simulink library "elementsLibrary"  (R2018a)
settings: Solver=VariableStepAuto  StartTime=0.0  StopTime=10.0  RelTol=1e-3
undefined symbols (not defined in the file): aerodynamics, ascent, avionics, environment, payload, propulsion, pvessel, recovery, rocket, sequencer
libraries: snippetLibrary x43, $bdroot x24, sharedutil x8, theirs_elementsLibrary x3, simulink_extras x1, aerolibutil x1
(part 4 of 4)

== system elementsLibrary/barrowmanExt/Coefficient of normal force/Body tube correction ==
  AOA : Inport
  Constant : Constant  Value=aerodynamics.K
  Constant1 : Constant  Value=aerodynamics.Ap
  Constant2 : Constant  Value=aerodynamics.Ar
  Divide : Product  Inputs=***/
  Sin : Trigonometry
  Square : Math  Operator=square  SaturateOnIntegerOverflow=on
  Cn_BodyCorrection : Outport
  wires:
  AOA/1 -> Sin/1
  Sin/1 -> Square/1
  Constant2/1 -> Divide/4
  Constant/1 -> Divide/1
  Constant1/1 -> Divide/2
  Square/1 -> Divide/3
  Divide/1 -> Cn_BodyCorrection/1

== system elementsLibrary/barrowmanExt/Coefficient of normal force/Cna Body Tube ==
  AOA : Inport
  Constant1 : Constant  Value=2
  Multiply : Product
  Subsystem : Subsystem
  Cna_nosecone : Outport
  wires:
  AOA/1 -> Subsystem/1(AOA)
  Subsystem/1(Correction) -> Multiply/2
  Constant1/1 -> Multiply/1
  Multiply/1 -> Cna_nosecone/1

== system elementsLibrary/barrowmanExt/Coefficient of normal force/Cna Fins ==
  AOA : Inport
  Mach : Inport  Port=2
  k1 : Inport  Port=3
  k2 : Inport  Port=4
  k3 : Inport  Port=5
  Constant : Constant  Value=aerodynamics.nf/2
  Constant1 : Constant  Value=aerodynamics.K_BF
  If : If  IfExpression=u1 <= 0.9  ElseIfExpressions=u1 >= 1.5
  Merge : Merge  Inputs=3
  Multiply : Product
  Multiply1 : Product
  Supersonic case : Subsystem  TreatAsAtomicUnit=on
  Transonic case : Subsystem  TreatAsAtomicUnit=on
  subsonic case : Subsystem  TreatAsAtomicUnit=on
  Cna_fins_w_FB_inter : Outport
  wires:
  Mach/1 -> Transonic case/1(Mach), subsonic case/1(Mach), If/1
  If/1 -> subsonic case/Action
  AOA/1 -> Supersonic case/1(AOA)
  k1/1 -> Supersonic case/2(k1)
  k2/1 -> Supersonic case/3(k2)
  k3/1 -> Supersonic case/4(k3)
  If/2 -> Supersonic case/Action
  If/3 -> Transonic case/Action
  Merge/1 -> Multiply/2
  Constant/1 -> Multiply/1
  subsonic case/1(Cna_1fin_subsonic) -> Merge/1
  Transonic case/1(Cna_1fin_Transonic) -> Merge/2
  Supersonic case/1(Cna_1fin_supersonic) -> Merge/3
  Constant1/1 -> Multiply1/1
  Multiply/1 -> Multiply1/2
  Multiply1/1 -> Cna_fins_w_FB_inter/1

== system elementsLibrary/barrowmanExt/Moment Coefficients from nosetip/Pitch Moment Coeff ==
  Xcp : Inport
  Cn : Inport  Port=2
  Constant : Constant  Value=aerodynamics.dn
  Divide : Product  Inputs=**/
  Cm_pitch_cp : Outport
  wires:
  Xcp/1 -> Divide/1
  Cn/1 -> Divide/2
  Constant/1 -> Divide/3
  Divide/1 -> Cm_pitch_cp/1

== system elementsLibrary/barrowmanExt/Moment Coefficients from nosetip/Subsystem ==
  Cm_pitch_cp : Inport
  Cn : Inport  Port=2
  Xcg : Inport  Port=3
  Constant : Constant  Value=aerodynamics.dn
  Divide : Product  Inputs=**/
  Subtract : Sum  Inputs=+-
  Cm_pitch_cg : Outport
  wires:
  Cn/1 -> Divide/1
  Xcg/1 -> Divide/2
  Constant/1 -> Divide/3
  Cm_pitch_cp/1 -> Subtract/1
  Divide/1 -> Subtract/2
  Subtract/1 -> Cm_pitch_cg/1

== system elementsLibrary/Ascentv1/Calculate Aero Coeffs & Center of Pressure/calculate ZAOA_cd/BaseCd ==
  Cd_fb : Inport
  Constant : Constant  Value=ascent.aerodynamics.dd
  Constant1 : Constant  Value=ascent.aerodynamics.db
  Constant2 : Constant  Value=3
  Divide : Product  Inputs=*/
  Divide1 : Product  Inputs=*/
  Gain : Gain  Gain=0.029
  Power : Math  Operator=pow  SaturateOnIntegerOverflow=on
  Sqrt : Sqrt  SaturateOnIntegerOverflow=on
  Cdb : Outport
  wires:
  Cd_fb/1 -> Sqrt/1
  Constant1/1 -> Divide/2
  Constant/1 -> Divide/1
  Divide/1 -> Power/1
  Constant2/1 -> Power/2
  Power/1 -> Divide1/1
  Sqrt/1 -> Divide1/2
  Divide1/1 -> Gain/1
  Gain/1 -> Cdb/1

== system elementsLibrary/Ascentv1/Calculate Aero Coeffs & Center of Pressure/calculate ZAOA_cd/FinsetCd ==
  Cf_f : Inport
  Add : Sum
  Constant : Constant  Value=ascent.aerodynamics.A_fp
  Constant1 : Constant  Value=ascent.aerodynamics.df
  Constant2 : Constant
  Constant3 : Constant  Value=ascent.aerodynamics.tf
  Constant4 : Constant  Value=ascent.aerodynamics.lm
  Divide : Product  Inputs=*/
  Divide1 : Product  Inputs=*/
  Gain : Gain  Gain=4
  Gain1 : Gain  Gain=pi
  Gain2 : Gain  Gain=2
  Gain3 : Gain  Gain=2
  Gain4 : Gain  Gain=ascent.aerodynamics.nf
  Multiply : Product  Inputs=3
  Square : Math  Operator=square  SaturateOnIntegerOverflow=on
  Cdf : Outport
  wires:
  Constant/1 -> Gain/1
  Constant1/1 -> Square/1
  Gain1/1 -> Divide/2
  Divide/1 -> Multiply/3
  Square/1 -> Gain1/1
  Cf_f/1 -> Gain2/1
  Constant2/1 -> Add/1
  Constant3/1 -> Divide1/1
  Constant4/1 -> Divide1/2
  Divide1/1 -> Gain3/1
  Gain3/1 -> Add/2
  Add/1 -> Multiply/2
  Gain2/1 -> Multiply/1
  Gain4/1 -> Divide/1
  Gain/1 -> Gain4/1
  Multiply/1 -> Cdf/1

== system elementsLibrary/Ascentv1/Calculate Aero Coeffs & Center of Pressure/calculate ZAOA_cd/ForebodyCd ==
  Cf_fb : Inport
  Add : Sum  Inputs=+++
  Add1 : Sum  Inputs=+++
  Constant : Constant
  Constant1 : Constant  Value=60
  Constant2 : Constant  Value=ascent.aerodynamics.lb/ascent.aerodynamics.db
  Constant3 : Constant  Value=ascent.aerodynamics.l_TR/ascent.aerodynamics.db
  Constant4 : Constant  Value=3
  Constant5 : Constant  Value=1-(ascent.aerodynamics.dd/ascent.aerodynamics.db)
  Constant6 : Constant  Value=ascent.aerodynamics.lc/ascent.aerodynamics.db
  Constant7 : Constant  Value=ascent.aerodynamics.ln/ascent.aerodynamics.db
  Constant8 : Constant  Value=ascent.aerodynamics.lb/ascent.aerodynamics.db
  Divide : Product  Inputs=/*
  Gain : Gain  Gain=0.0025
  Gain1 : Gain  Gain=2
  Gain2 : Gain  Gain=2.7
  Gain3 : Gain  Gain=4
  Multiply : Product  Inputs=3
  Multiply1 : Product
  Power : Math  Operator=pow  SaturateOnIntegerOverflow=on
  Cd_fb : Outport
  wires:
  Multiply/1 -> Cd_fb/1
  Cf_fb/1 -> Multiply/1
  Add/1 -> Multiply/2
  Add1/1 -> Multiply/3
  Constant/1 -> Add/3
  Divide/1 -> Add/1
  Constant1/1 -> Divide/2
  Gain/1 -> Add/2
  Constant2/1 -> Gain/1
  Power/1 -> Divide/1
  Constant3/1 -> Power/1
  Constant4/1 -> Power/2
  Gain1/1 -> Add1/1
  Multiply1/1 -> Gain1/1
  Constant5/1 -> Multiply1/1
  Constant6/1 -> Multiply1/2
  Gain2/1 -> Add1/2
  Gain3/1 -> Add1/3
  Constant7/1 -> Gain2/1
  Constant8/1 -> Gain3/1

== system elementsLibrary/Ascentv1/Calculate Aero Coeffs & Center of Pressure/calculate ZAOA_cd/InterferenceCd ==
  Cf_f : Inport
  Add : Sum
  Constant : Constant  Value=ascent.aerodynamics.A_fp - ascent.aerodynamics.A_fe
  Constant1 : Constant  Value=ascent.aerodynamics.df
  Constant2 : Constant
  Constant3 : Constant  Value=ascent.aerodynamics.tf
  Constant4 : Constant  Value=ascent.aerodynamics.lm
  Divide : Product  Inputs=*/
  Divide1 : Product  Inputs=*/
  Gain : Gain  Gain=4
  Gain1 : Gain  Gain=pi
  Gain2 : Gain  Gain=2
  Gain3 : Gain  Gain=2
  Gain4 : Gain  Gain=ascent.aerodynamics.nf
  Multiply : Product  Inputs=3
  Square : Math  Operator=square  SaturateOnIntegerOverflow=on
  Cdi : Outport
  wires:
  Add/1 -> Multiply/2
  Multiply/1 -> Cdi/1
  Square/1 -> Gain1/1
  Constant1/1 -> Square/1
  Constant/1 -> Gain/1
  Gain1/1 -> Divide/2
  Divide/1 -> Multiply/3
  Constant2/1 -> Add/1
  Gain4/1 -> Divide/1
  Constant4/1 -> Divide1/2
  Divide1/1 -> Gain3/1
  Gain3/1 -> Add/2
  Gain2/1 -> Multiply/1
  Constant3/1 -> Divide1/1
  Gain/1 -> Gain4/1
  Cf_f/1 -> Gain2/1

== system elementsLibrary/Ascentv2/Rotational/Inertia_Matrix /parallelAxisTheo_restricted ==
  emptyInertia : Inport
  motorInertias : Inport  Port=2
  propellantMass : Inport  Port=3
  rocketEmptyXcg : Inport  Port=4
  motorProperties : Inport  Port=5
  Add : Sum
  Add1 : Sum
  Add2 : Sum
  Bus Selector : BusSelector  OutputSignals=x_gm_B,x_cg_B
  Constant{1..7} (7 alike) : Constant  Value=0
  Create 3x3 Matrix : sharedutil/Create 3x3 Matrix  aMode=aMode
  Multiply : Product
  Square : Math  Operator=square  SaturateOnIntegerOverflow=on
  Subtract : Sum  Inputs=+-
  J_rocket : Outport
  wires:
  Constant6/1 -> Create 3x3 Matrix/7
  Constant7/1 -> Create 3x3 Matrix/4
  Create 3x3 Matrix/1 -> Add1/2
  Constant4/1 -> Create 3x3 Matrix/6
  Constant5/1 -> Create 3x3 Matrix/8
  Constant1/1 -> Create 3x3 Matrix/2
  Multiply/1 -> Create 3x3 Matrix/5, Create 3x3 Matrix/9
  Constant2/1 -> Create 3x3 Matrix/3
  Add/1 -> J_rocket/1  "J_equivalent"
  Add1/1 -> Add/2
  propellantMass/1 -> Multiply/1
  motorInertias/1 -> Add1/1
  emptyInertia/1 -> Add/1
  rocketEmptyXcg/1 -> Subtract/2
  Constant3/1 -> Create 3x3 Matrix/1
  Subtract/1 -> Square/1
  Square/1 -> Multiply/2
  Bus Selector/1 -> Add2/1  "<x_gm_B>"
  Bus Selector/2 -> Add2/2  "<x_cg_B>"
  Add2/1 -> Subtract/1
  motorProperties/1 -> Bus Selector/1

== system elementsLibrary/HREV1/Chamber_Ballistics/calc_chamber_params/If Action Subsystem ==
  In1 : Inport
  Action Port : ActionPort  ActionType=then
  Out1 : Outport
  wires:
  In1/1 -> Out1/1

== system elementsLibrary/HREV1/Chamber_Ballistics/calc_chamber_params/If Action Subsystem1 ==
  In1 : Inport
  Action Port : ActionPort  ActionType=else
  Out1 : Outport
  wires:
  In1/1 -> Out1/1

== system elementsLibrary/HREV1/Chamber_Ballistics/calc_chamber_params/calc_Tc ==
  OF_ratio : Inport
  Add : Sum  Inputs=+++++
  Constant : Constant  Value=-15.854
  Constant1 : Constant  Value=4
  Constant2 : Constant  Value=314.21
  Constant3 : Constant  Value=3
  Constant4 : Constant  Value=-2334.4
  Constant5 : Constant  Value=2
  Constant6 : Constant  Value=-5742.5
  Constant7 : Constant  Value=7623.5
  Multiply{,1..3} (4 alike) : Product
  Power1 : Math  Operator=pow  SaturateOnIntegerOverflow=on
  Power2 : Math  Operator=pow  SaturateOnIntegerOverflow=on
  Power3 : Math  Operator=pow  SaturateOnIntegerOverflow=on
  Saturation : Saturate  UpperLimit=10000  LowerLimit=273.15
  Tc : Outport
  wires:
  OF_ratio/1 -> Power3/1, Power1/1, Power2/1, Multiply3/2
  Multiply/1 -> Add/1
  Multiply1/1 -> Add/2
  Multiply2/1 -> Add/3
  Multiply3/1 -> Add/4
  Constant6/1 -> Add/5
  Power3/1 -> Multiply2/2
  Power2/1 -> Multiply/2
  Power1/1 -> Multiply1/2
  Constant/1 -> Multiply/1
  Constant1/1 -> Power2/2
  Constant2/1 -> Multiply1/1
  Constant3/1 -> Power1/2
  Constant4/1 -> Multiply2/1
  Constant5/1 -> Power3/2
  Constant7/1 -> Multiply3/1
  Saturation/1 -> Tc/1
  Add/1 -> Saturation/1

== system elementsLibrary/HREV1/Chamber_Ballistics/calc_mdot_fuel/calc_OF ==
  mdot_fuel : Inport
  mdot_oxi : Inport  Port=2
  Constant : Constant  Value=0
  Divide : Product  Inputs=*/
  If : If
  If Action Subsystem : Subsystem  TreatAsAtomicUnit=on
  If Action Subsystem1 : Subsystem  TreatAsAtomicUnit=on
  Merge : Merge
  OF_ratio : Outport
  wires:
  mdot_oxi/1 -> Divide/1
  mdot_fuel/1 -> If/1, Divide/2
  If Action Subsystem1/1(Out1) -> Merge/2
  Constant/1 -> If Action Subsystem1/1(In1)
  If/2 -> If Action Subsystem1/Action
  If Action Subsystem/1(Out1) -> Merge/1
  If/1 -> If Action Subsystem/Action
  Merge/1 -> OF_ratio/1
  Divide/1 -> If Action Subsystem/1(In1)

== system elementsLibrary/HREV1/Chamber_Ballistics/calc_mdot_fuel/calc_massFlux_oxi ==
  Dp : Inport
  mdot_oxi : Inport  Port=2
  Divide : Product  Inputs=*/
  Gain : Gain  Gain=4
  Multiply : Product
  Pi : Constant  Value=pi
  Square : Math  Operator=square  SaturateOnIntegerOverflow=on
  Gox : Outport
  wires:
  Divide/1 -> Gox/1
  Dp/1 -> Square/1
  Multiply/1 -> Divide/2
  Square/1 -> Multiply/2
  Pi/1 -> Multiply/1
  Gain/1 -> Divide/1
  mdot_oxi/1 -> Gain/1

== system elementsLibrary/HREV1/Chamber_Ballistics/calc_mdot_fuel/calc_mdot_fuel ==
  rdot_fuel : Inport
  Dp : Inport  Port=2
  rho_oxi : Inport  Port=3
  Add : Sum  Inputs=-+
  Constant : Constant  Value=0
  Constant1 : Constant  Value=propulsion.initMassFuel
  Integrator : Integrator
  LessThanOrEqual : RelationalOperator  Operator=>  OutDataTypeStr=boolean  RndMeth=Simplest
  Multiply : Product  Inputs=5
  Multiply1 : Product
  Pi : Constant  Value=pi
  grainL : Constant  Value=propulsion.Lfg
  mdot_fuel : Outport
  massFuel : Outport  Port=2
  wires:
  Multiply/1 -> Multiply1/1
  rho_oxi/1 -> Multiply/1
  Pi/1 -> Multiply/2
  rdot_fuel/1 -> Multiply/5
  Dp/1 -> Multiply/3
  grainL/1 -> Multiply/4
  Integrator/1 -> Add/1
  Constant1/1 -> Add/2
  Add/1 -> massFuel/1, LessThanOrEqual/1
  Constant/1 -> LessThanOrEqual/2
  LessThanOrEqual/1 -> Multiply1/2
  Multiply1/1 -> Integrator/1, mdot_fuel/1

== system elementsLibrary/HREV1/Chamber_Ballistics/calc_mdot_fuel/calc_rdot_fuel ==
  Gox : Inport
  Multiply : Product
  Power : Math  Operator=pow  SaturateOnIntegerOverflow=on
  a : Constant  Value=propulsion.a
  mm/s_to_m/s : Gain  Gain=0.001
  n : Constant  Value=propulsion.n
  rdot_fuel : Outport
  wires:
  Multiply/1 -> mm/s_to_m/s/1
  Power/1 -> Multiply/2
  Gox/1 -> Power/1
  n/1 -> Power/2
  a/1 -> Multiply/1
  mm/s_to_m/s/1 -> rdot_fuel/1

== system elementsLibrary/SingleChute/Rotational Motion/equations of rotational motion/invInertia_Matrix_P ==
  Constant : Constant  Value=recovery.inertiaMatP(1,1)
  Constant1 : Constant  Value=recovery.inertiaMatP(1,2)
  Constant2 : Constant  Value=recovery.inertiaMatP(1,3)
  Constant3 : Constant  Value=recovery.inertiaMatP(2,1)
  Constant4 : Constant  Value=recovery.inertiaMatP(2,2)
  Constant5 : Constant  Value=recovery.inertiaMatP(2,3)
  Constant6 : Constant  Value=recovery.inertiaMatP(3,1)
  Constant7 : Constant  Value=recovery.inertiaMatP(3,2)
  Constant8 : Constant  Value=recovery.inertiaMatP(3,3)
  Create 3x3 Matrix : sharedutil/Create 3x3 Matrix  aMode=aMode
  inverse_3x3 : snippetLibrary/mathSnippets/inverse_3x3
  invInerMat : Outport
  inerMat : Outport  Port=2
  wires:
  Constant3/1 -> Create 3x3 Matrix/4
  Constant8/1 -> Create 3x3 Matrix/9
  Create 3x3 Matrix/1 -> inerMat/1, inverse_3x3/1
  Constant4/1 -> Create 3x3 Matrix/5
  inverse_3x3/1 -> invInerMat/1
  Constant/1 -> Create 3x3 Matrix/1
  Constant5/1 -> Create 3x3 Matrix/6
  Constant7/1 -> Create 3x3 Matrix/8
  Constant1/1 -> Create 3x3 Matrix/2
  Constant2/1 -> Create 3x3 Matrix/3
  Constant6/1 -> Create 3x3 Matrix/7

== system elementsLibrary/SingleChute/Rotational Motion/equations of rotational motion/invInertia_Matrix_R ==
  Constant : Constant  Value=recovery.inertiaMatR(1,1)
  Constant1 : Constant  Value=recovery.inertiaMatR(1,2)
  Constant2 : Constant  Value=recovery.inertiaMatR(1,3)
  Constant3 : Constant  Value=recovery.inertiaMatR(2,1)
  Constant4 : Constant  Value=recovery.inertiaMatR(2,2)
  Constant5 : Constant  Value=recovery.inertiaMatR(2,3)
  Constant6 : Constant  Value=recovery.inertiaMatR(3,1)
  Constant7 : Constant  Value=recovery.inertiaMatR(3,2)
  Constant8 : Constant  Value=recovery.inertiaMatR(3,3)
  Create 3x3 Matrix : sharedutil/Create 3x3 Matrix  aMode=aMode
  inverse_3x3 : snippetLibrary/mathSnippets/inverse_3x3
  invInerMat : Outport
  inerMat : Outport  Port=2
  wires:
  inverse_3x3/1 -> invInerMat/1
  Constant4/1 -> Create 3x3 Matrix/5
  Constant2/1 -> Create 3x3 Matrix/3
  Constant7/1 -> Create 3x3 Matrix/8
  Constant/1 -> Create 3x3 Matrix/1
  Constant1/1 -> Create 3x3 Matrix/2
  Constant5/1 -> Create 3x3 Matrix/6
  Constant3/1 -> Create 3x3 Matrix/4
  Constant6/1 -> Create 3x3 Matrix/7
  Constant8/1 -> Create 3x3 Matrix/9
  Create 3x3 Matrix/1 -> inerMat/1, inverse_3x3/1

== system elementsLibrary/barrowmanExt/Center of Pressure/Calc Xcp fins/If Action Subsystem ==
  Action Port : ActionPort
  Constant : Constant  Value=aerodynamics.Xcp_fins
  Xcp_fins_subMach0.5 : Outport
  wires:
  Constant/1 -> Xcp_fins_subMach0.5/1

== system elementsLibrary/barrowmanExt/Center of Pressure/Calc Xcp fins/If Action Subsystem1 ==
  Mach : Inport
  Action Port : ActionPort
  Add : Sum
  Calc Beta : Subsystem
  Constant : Constant  Value=aerodynamics.AsRa
  Constant1 : Constant  Value=aerodynamics.lm
  Constant2 : Constant  Value=0.67
  Constant3 : Constant  Value=2*aerodynamics.AsRa
  Constant4 : Constant
  Constant5 : Constant  Value=aerodynamics.macLead
  Divide : Product  Inputs=**/
  Multiply : Product
  Multiply1 : Product
  Subtract : Sum  Inputs=+-
  Subtract1 : Sum  Inputs=+-
  Xcp_fins_above2 : Outport
  wires:
  Mach/1 -> Calc Beta/1(Mach)
  Calc Beta/1(Beta) -> Multiply1/1, Multiply/2
  Constant/1 -> Multiply/1
  Multiply/1 -> Subtract/1
  Constant2/1 -> Subtract/2
  Constant3/1 -> Multiply1/2
  Multiply1/1 -> Subtract1/1
  Constant4/1 -> Subtract1/2
  Subtract1/1 -> Divide/3
  Subtract/1 -> Divide/2
  Constant1/1 -> Divide/1
  Divide/1 -> Add/2
  Constant5/1 -> Add/1
  Add/1 -> Xcp_fins_above2/1

== system elementsLibrary/barrowmanExt/Center of Pressure/Calc Xcp fins/If Action Subsystem2 ==
  Mach : Inport
  Action Port : ActionPort
  Add : Sum
  Constant : Constant  Value=aerodynamics.macLead
  Polynomial : Polyval  Coefs=aerodynamics.finXcpPoly
  Xcp_finsTrans : Outport
  wires:
  Mach/1 -> Polynomial/1
  Polynomial/1 -> Add/1
  Constant/1 -> Add/2
  Add/1 -> Xcp_finsTrans/1

== system elementsLibrary/barrowmanExt/Coefficent of drag 0 AOA/Pressure Drag Coefficient/Fin Pressure Drag ==
  stagD : Inport
  baseD : Inport  Port=2
  Add : Sum
  Atan2 : Trigonometry  Operator=atan2
  Constant : Constant  Value=aerodynamics.lw
  Constant1 : Constant  Value=aerodynamics.nf
  Constant2 : Constant  Value=aerodynamics.tf
  Constant3 : Constant  Value=aerodynamics.Ar
  Constant4 : Constant  Value=aerodynamics.lw
  Constant5 : Constant  Value=aerodynamics.ls
  Cos : Trigonometry  Operator=cos
  Divide : Product  Inputs=*/
  Multiply : Product
  Multiply1 : Product  Inputs=4
  Square : Math  Operator=square  SaturateOnIntegerOverflow=on
  finPD : Outport
  wires:
  Square/1 -> Multiply/1
  Cos/1 -> Square/1
  Atan2/1 -> Cos/1
  Constant4/1 -> Atan2/2
  Constant5/1 -> Atan2/1
  Divide/1 -> finPD/1
  Constant3/1 -> Divide/2
  Multiply1/1 -> Divide/1
  Constant2/1 -> Multiply1/4
  Constant1/1 -> Multiply1/3
  Constant/1 -> Multiply1/2
  Add/1 -> Multiply1/1
  Multiply/1 -> Add/1
  baseD/1 -> Add/2
  stagD/1 -> Multiply/2

== system elementsLibrary/barrowmanExt/Coefficient of normal force/Cna Body Tube/Subsystem ==
  AOA : Inport
  If : If  IfExpression=u1 < 0.0001
  If Action Subsystem : Subsystem  TreatAsAtomicUnit=on
  If Action Subsystem1 : Subsystem  TreatAsAtomicUnit=on
  Merge : Merge
  Correction : Outport
  wires:
  AOA/1 -> If Action Subsystem1/1(AOA), If/1
  If/1 -> If Action Subsystem/Action
  If/2 -> If Action Subsystem1/Action
  If Action Subsystem/1(Correction) -> Merge/1
  If Action Subsystem1/1(Correction) -> Merge/2
  Merge/1 -> Correction/1

== system elementsLibrary/barrowmanExt/Coefficient of normal force/Cna Fins/Supersonic case ==
  AOA : Inport
  k1 : Inport  Port=2
  k2 : Inport  Port=3
  k3 : Inport  Port=4
  Action Port : ActionPort
  Single Fin Cna Supersonic : Subsystem
  Cna_1fin_supersonic : Outport
  wires:
  AOA/1 -> Single Fin Cna Supersonic/1(AOA)
  k1/1 -> Single Fin Cna Supersonic/2(k1)
  k3/1 -> Single Fin Cna Supersonic/4(k3)
  k2/1 -> Single Fin Cna Supersonic/3(k2)
  Single Fin Cna Supersonic/1(Cna_1fin_supersonic) -> Cna_1fin_supersonic/1

== system elementsLibrary/barrowmanExt/Coefficient of normal force/Cna Fins/Transonic case ==
  Mach : Inport
  Action Port : ActionPort
  1-D Lookup Table : Lookup_n-D  NumberOfTableDimensions=1  BreakpointsForDimension1=aerodynamics.transCnaFinsBreakpoints  Table=aerodynamics.transCnaFins  InternalRulePriority=Speed  RndMeth=Simplest  InputSameDT=on
  Cna_1fin_Transonic : Outport
  wires:
  Mach/1 -> 1-D Lookup Table/1
  1-D Lookup Table/1 -> Cna_1fin_Transonic/1

== system elementsLibrary/barrowmanExt/Coefficient of normal force/Cna Fins/subsonic case ==
  Mach : Inport
  Action Port : ActionPort
  Single Fin Cna subsonic : Subsystem
  Cna_1fin_subsonic : Outport
  wires:
  Mach/1 -> Single Fin Cna subsonic/1(Mach)
  Single Fin Cna subsonic/1(Cna_1Fin_subsonic) -> Cna_1fin_subsonic/1

== system elementsLibrary/HREV1/Chamber_Ballistics/calc_mdot_fuel/calc_OF/If Action Subsystem ==
  In1 : Inport
  Action Port : ActionPort  ActionType=then
  Out1 : Outport
  wires:
  In1/1 -> Out1/1

== system elementsLibrary/HREV1/Chamber_Ballistics/calc_mdot_fuel/calc_OF/If Action Subsystem1 ==
  In1 : Inport
  Action Port : ActionPort  ActionType=else
  Out1 : Outport
  wires:
  In1/1 -> Out1/1

== system elementsLibrary/barrowmanExt/Center of Pressure/Calc Xcp fins/If Action Subsystem1/Calc Beta ==
  Mach : Inport
  Abs : Abs
  Constant : Constant
  Sqrt : Sqrt  SaturateOnIntegerOverflow=on
  Square : Math  Operator=square  SaturateOnIntegerOverflow=on
  Subtract : Sum  Inputs=+-
  Beta : Outport
  wires:
  Mach/1 -> Square/1
  Constant/1 -> Subtract/2
  Square/1 -> Subtract/1
  Subtract/1 -> Abs/1
  Abs/1 -> Sqrt/1
  Sqrt/1 -> Beta/1

== system elementsLibrary/barrowmanExt/Coefficient of normal force/Cna Body Tube/Subsystem/If Action Subsystem ==
  Action Port : ActionPort
  Constant : Constant
  Correction : Outport
  wires:
  Constant/1 -> Correction/1

== system elementsLibrary/barrowmanExt/Coefficient of normal force/Cna Body Tube/Subsystem/If Action Subsystem1 ==
  AOA : Inport
  Action Port : ActionPort
  Divide : Product  Inputs=*/
  Sin : Trigonometry
  Correction : Outport
  wires:
  AOA/1 -> Divide/2, Sin/1
  Sin/1 -> Divide/1
  Divide/1 -> Correction/1

== system elementsLibrary/barrowmanExt/Coefficient of normal force/Cna Fins/Supersonic case/Single Fin Cna Supersonic ==
  AOA : Inport
  k1 : Inport  Port=2
  k2 : Inport  Port=3
  k3 : Inport  Port=4
  Add : Sum  Inputs=+++
  Constant : Constant  Value=aerodynamics.A_fwt/aerodynamics.Ar
  Multiply : Product
  Multiply1 : Product
  Multiply2 : Product
  Square : Math  Operator=square  SaturateOnIntegerOverflow=on
  Cna_1fin_supersonic : Outport
  wires:
  AOA/1 -> Square/1, Multiply/2
  Square/1 -> Multiply1/1
  k3/1 -> Multiply1/2
  k2/1 -> Multiply/1
  Multiply1/1 -> Add/3
  Multiply/1 -> Add/2
  k1/1 -> Add/1
  Add/1 -> Multiply2/2
  Constant/1 -> Multiply2/1
  Multiply2/1 -> Cna_1fin_supersonic/1

== system elementsLibrary/barrowmanExt/Coefficient of normal force/Cna Fins/subsonic case/Single Fin Cna subsonic ==
  Mach : Inport
  Add : Sum
  Add1 : Sum
  Constant : Constant  Value=2
  Constant1 : Constant  Value=aerodynamics.ls
  Constant2 : Constant  Value=aerodynamics.Ar
  Constant3 : Constant  Value=aerodynamics.A_fwt
  Constant4 : Constant  Value=aerodynamics.sweepAgl
  Constant5 : Constant
  Constant6 : Constant
  Constant7 : Constant  VectorParams1D=off  SampleTime=-1
  Cos : Trigonometry  Operator=cos
  Divide : Product  Inputs=***/
  Divide1 : Product  Inputs=**//
  Divide2 : Product  Inputs=*/
  Pi : Constant  Value=pi
  Sqrt : Sqrt  SaturateOnIntegerOverflow=on
  Sqrt1 : Sqrt  SaturateOnIntegerOverflow=on
  Square : Math  Operator=square  SaturateOnIntegerOverflow=on
  Square1 : Math  Operator=square  SaturateOnIntegerOverflow=on
  Square2 : Math  Operator=square  SaturateOnIntegerOverflow=on
  Subtract : Sum  Inputs=+-
  Cna_1Fin_subsonic : Outport
  wires:
  Constant/1 -> Divide/1
  Pi/1 -> Divide/2
  Square/1 -> Divide1/1, Divide/3
  Constant1/1 -> Square/1
  Constant2/1 -> Divide/4
  Constant6/1 -> Subtract/1
  Mach/1 -> Square1/1
  Square1/1 -> Subtract/2
  Subtract/1 -> Sqrt1/1
  Sqrt1/1 -> Divide1/2
  Constant3/1 -> Divide1/3
  Cos/1 -> Divide1/4
  Constant4/1 -> Cos/1
  Divide1/1 -> Square2/1
  Square2/1 -> Add1/2
  Constant5/1 -> Add1/1
  Add1/1 -> Sqrt/1
  Constant7/1 -> Add/1
  Sqrt/1 -> Add/2
  Add/1 -> Divide2/2
  Divide/1 -> Divide2/1
  Divide2/1 -> Cna_1Fin_subsonic/1

== matlab function elementsLibrary/AvionicsCharacterization/MATLAB Function ==
  data: posZ_E input; airbrakeCmdAngle output; velMag input; velZ_E input; thurstMag_B input; deploy1 output; deploy2 output; airbrakeDeploySpeed input; airbrakeDeployCmd input; descentTwoDeployAltitude input; prevDeploy1 input; prevDeploy2 input
function [airbrakeCmdAngle, deploy1, deploy2]= avionicsChLogic(posZ_E, velMag, velZ_E,...
                                                               thurstMag_B,...
                                                               airbrakeDeploySpeed,...
                                                               airbrakeDeployCmd,...
                                                               descentTwoDeployAltitude,...
                                                               prevDeploy1,...
                                                               prevDeploy2)
    
    airbrakeCmdAngle = 0;
    
    deploy1 = prevDeploy1;
    deploy2 = prevDeploy2;
    
    if(prevDeploy1 == 0 && velZ_E < 0 && velMag < 0)
        deploy1 = 1;   
    end
    
    if(prevDeploy2 == 0 && velZ_E < 0 && velMag < 0 && posZ_E <= descentTwoDeployAltitude)
        deploy2 = 1;
    end

    if(thurstMag_B == 0 && velZ_E > 0 && velMag <= airbrakeDeploySpeed)
        airbrakeCmdAngle = airbrakeDeployCmd;
    end
    
end

== matlab function elementsLibrary/FSv1/MATLAB Function ==
  data: towerLen input; flightState output; posMag input; posX_E input; posY_E input; posZ_E input; roll input; pitch input; yaw input; velX_E input; velY_E input; velZ_E input; descentOneDeploy input; descentTwoDeploy input; thurstMag_B input; prevFlightState input; stop output
function [flightState, stop]= sequencingLogic(towerLen, posMag, posX_E, posY_E, posZ_E,...
                                              roll, pitch, yaw, velX_E, velY_E, velZ_E,...
                                              descentOneDeploy, descentTwoDeploy,...
                                              thurstMag_B, prevFlightState)

    stop = false;
    
    if(velZ_E < 0 && (prevFlightState == 3 || prevFlightState == 2))
        stop = true;
    end
    
    if(posMag <= towerLen && thurstMag_B == 0 && prevFlightState == 0)
        
        flightState = 0;
        
    elseif(posMag <= towerLen && thurstMag_B ~= 0 && (prevFlightState == 0 || prevFlightState == 1))
        
        flightState = 1;
        
    elseif(posMag <= towerLen && thurstMag_B == 0 && prevFlightState == 5)
        
        flightState = 6;
        stop = true;
        
    elseif(posMag > towerLen && thurstMag_B == 0)
        
        flightState = 3;
        
        if(descentOneDeploy)
            flightState = 4;
        end
        
        if(descentOneDeploy && descentTwoDeploy)
            flightState = 5;
        end

    elseif(posMag > towerLen && thurstMag_B ~= 0)
        
        flightState = 2;
        
    else
        
        flightState = -1;
        
    end
    
end

== matlab function elementsLibrary/Ascentv1/Calculate Aero Coeffs & Center of Pressure/calcAeroCoeffs ==
  data: mach input; cd input; AOA input; aeroRollAngle input; Va input; Cn_B output size=1; Ca_B output size=1; Cy_B output size=1; Cz_B output size=1; Xcp output size=1; Cm_B output size=1; lw parameter; ls parameter; lr parameter; lt parameter; Ar parameter; A_fwt parameter; Ap parameter; df parameter; nf parameter; dn parameter; du parameter; ln parameter; lb parameter; CNalpha_nose parameter; Xcp_nose parameter; Xcp_body parameter; Xcp_fins parameter; Xf parameter; CN_body output; CN_nose output; CN_fins output
function [Cn_B, Ca_B, Cy_B, Cz_B, Xcp, Cm_B, CN_body, CN_nose, CN_fins] = calcAeroCeoffs(mach, cd, AOA, aeroRollAngle, Va,...
                                                                                         lw, ls, lr, lt, Ar, A_fwt, Ap, df,...
                                                                                         nf, dn, du, ln, lb, CNalpha_nose,...
                                                                                         Xcp_nose, Xcp_body, Xcp_fins, Xf)
    
                                                          
    Cn_B = 0;
    Ca_B = 0;
    Cy_B = 0; 
    Cz_B = 0;
    Xcp = 0;
    Cm_B = 0;
       
    STALL_ANGLE = 20*(pi/180);
    
%     if(AOA >= 1*(pi/180))
%         AOA = 1*(pi/180);        
%     end
    
    aoa_min = min([AOA, pi - AOA, STALL_ANGLE]);
    aoa_min2 = min([AOA, STALL_ANGLE]);
    
    if(mach <= 0.8)
        beta = sqrt(1 - mach^2);
    elseif(mach > 0.8 && mach <= 1.1)
        beta = sqrt(1 - 0.8^2);
    else
        beta = sqrt(mach^2 - 1);
    end
    
    %if (mach < 1)
        gamma = atan2(lw+((lt-lr)/2), ls);
        CNalpha_1fin = ((2*pi*(ls)^2)/Ar)/(1 + sqrt(1 + ((beta*ls^2)/(A_fwt*cos(gamma)))^2));
    %else
    %    k = 1.4;
    %    k1 = 2/beta;
    %    k2 = ((k+1)*(mach^4)-4*(beta^2))/(4*(beta^4));
    %    k3 = (((k+1)*(mach^8))+((2*(k^2)-7*k-5)*(mach^6))+(10*(k+1)*(mach^4))+(8))/(6*(beta^7));
    %    CNalpha_1fin = (A_fwt/2)*(k1+(k2*aoa_min)+(k3*((aoa_min)^3)));
    %end

    % Cna & Xcp
    CNalpha_nose = CNalpha_nose*sinc(AOA);
    CNalpha_body = 0;
    CNalpha_fins = (1 + ((df/2)/(ls + (df/2))))*(nf/2)*CNalpha_1fin; %(1 + ((df/2)/(ls + (df/2))))*(nf/2)*CNalpha_1fin;
    
    Xcp_n = Xcp_nose;
    Xcp_b = 0;
    Xcp_f = Xcp_fins;
    
    % Lift Corrections
    mul = 1;
    if(mach < 0.05 && AOA > pi/4)
        mul = (mach/0.05)^2;
    end
   
    Cnal_nose = mul*1.1*(((dn*ln)/2)/Ar)*sin(AOA)*sinc(AOA);
    Cnal_body = mul*1.1*(Ap/Ar)*sin(AOA)*sinc(AOA);
    
    Xcpl_nose = (5/8)*ln;
    Xcpl_body = 0.5*lb;
    
    % Applications
    
    if(Cnal_nose+CNalpha_nose < 0.00000001^2)
        Xcpn = (Xcp_n+Xcpl_nose)/2;
        Cna_nose = 0;
    else
        Xcpn = (Xcp_n*CNalpha_nose+Xcpl_nose*Cnal_nose)/(Cnal_nose+CNalpha_nose);
        Cna_nose = Cnal_nose+CNalpha_nose;
    end
    
    CN_nose = Cna_nose*AOA;
    
    Xcpb = Xcpl_body;
    Cna_body = Cnal_body;
    CN_body = Cna_body*AOA;
    
    Xcpf = Xcp_f;
    Cna_fins = CNalpha_fins;
    CN_fins = Cna_fins*aoa_min2;
    
    CNa_total = Cna_nose + Cna_body + Cna_fins;
    CN_total = CN_nose + CN_body + CN_fins;
    
    Cn_B = CN_total;

    Xcpb = Xcpb + ln;
    Xcpf = Xcpf + Xf;
    
    Cm_body = CN_body*(Xcpb/dn);
    Cm_fins = CN_fins*(Xcpf/dn);
    Cm_nose = CN_nose*(Xcpn/dn);
    
    Cm_B = Cm_body + Cm_fins + Cm_nose;
    
    if(CNa_total < 0.00000001^2)
        Xcp = (Xcpn + Xcpb + Xcpf)/3;
        CNa_total = 0;
    else
        Xcp = (Xcpn*Cna_nose + Xcpb*Cna_body + Xcpf*Cna_fins)/CNa_total;
    end
    
    Ca_B = 1.3*cd*cos(AOA);
    Cy_B = 0;%Cn_B*sin(aeroRollAngle);
    Cz_B = 0;%Cn_B*cos(aeroRollAngle);
    
%     CNalpha_total = CNalpha_nose + CNalpha_body + CNalpha_fins;
%     
%     Cma_nose = ((pi*ln)/3)*((dn/2)^2);
%     Cma_body = ((pi*lb)/3)*(((dn/2)^2) + ((dn/2)*(du/2)) + ((du/2)*2));
%     Cma_total = Cma_nose + Cma_body;
%     
%     Xcp_n = (Cma_nose/CNalpha_nose)*dn;
    
%     if(CNalpha_body ~= 0)
%         Xcp_b = Xcp_body + (Cma_body/CNalpha_body)*dn; %(Cma_body/CNalpha_body)*ln;
%     else
%         Xcp_b = Xcp_body;
%     end
%     
%     Xcp = ((Xcp_n*CNalpha_nose) + (Xcp_b*CNalpha_body) + (Xcp_f*CNalpha_fins))/CNalpha_total;
%     
%     Cn_B = CNalpha_total*AOA;
%     Cm_B = Cma_total*AOA;
%     
%     
end

== matlab function elementsLibrary/Ascentv1/Rotation/momentDamping/calcMomentDamping ==
  data: Mx_damp output; My_damp output; Mz_damp output; Va input; angVel input; mach input; density_atm input; xcg input; X_finset input; ct input; cr input; rt input; s input; w input; l_TR input; l_ref input; A_ref input; Deq input; numFins input
function [Mx_damp, My_damp, Mz_damp]= calcMomentDamping(Va, angVel, mach, density_atm, xcg, X_finset, ct, cr, rt, s, w, l_TR, l_ref, A_ref, Deq, numFins)

% if(Va > 0)
%     if(mach <= 1)
%         beta = sqrt(1 - mach^2);
%         cld = ((2*numFins*pi*angVel(1))/(beta*A_ref*l_ref*Va))*(((cr+ct)/(2))*(rt^2)*(s) +...
%                                                                 ((cr+2*ct)/(3))*(rt)*(s^2) +...
%                                                                 ((cr+3*ct)/(12))*(s^3));
%     else
%         cld = ((numFins)/(A_ref*l_ref))*(((cr+ct)/(2))*(rt^2)*(s) +...
%                                          ((cr+2*ct)/(3))*(rt)*(s^2) +...
%                                          ((cr+3*ct)/(12))*(s^3));
%     end
% 
%     X_fins = abs(X_finset-xcg);
% 
%     cmq_fuselage = ((1.1*Deq*(xcg^4 + (l_TR - xcg)^4))/(4*l_ref*A_ref))*(angVel(2)/Va)^2;
%     cmq_finset = ((0.6*numFins*((s*(cr+ct))/2)*(X_fins+(w/2)+((cr+ct)/4))^2)/(l_ref*A_ref))*(angVel(2)/Va)^2;
% 
%     cnq_fuselage = ((1.1*Deq*(xcg^4 + (l_TR - xcg)^4))/(4*l_ref*A_ref))*(angVel(3)/Va)^2;
%     cnq_finset = ((0.6*numFins*((s*(cr+ct))/2)*(X_fins+(w/2)+((cr+ct)/4))^2)/(l_ref*A_ref))*(angVel(3)/Va)^2;
% 
%     Mx_damp = (0.5)*cld*density_atm*A_ref*l_ref*Va^2;
%     My_damp = (0.5)*(cmq_fuselage+cmq_finset)*density_atm*A_ref*l_ref*Va^2;
%     Mz_damp = (0.5)*(cnq_fuselage+cnq_finset)*density_atm*A_ref*l_ref*Va^2;
% else
%     Mx_damp = 0;
%     My_damp = 0;
%     Mz_damp = 0;
% end

Mx_damp = 0;
My_damp = 0;
Mz_damp = 0;

end

== matlab function elementsLibrary/Ascentv1/Calculate Aero Coeffs & Center of Pressure/calculate AOA & Side Slip/calcAoA ==
  data: Va input; alpha output; phiA output
function [alpha, phiA] = calcAOA(Va)

rollAxis = [1;...
            0;...
            0];

lateralMagnitude = sqrt((Va(2))^2 + (Va(3))^2);
VaMagnitude = (sqrt((Va(1))^2 + (Va(2))^2 + (Va(3))^2));         
VaNorm = Va/VaMagnitude;

if(VaMagnitude > 0.01)
    %alpha = acos(dot(rollAxis, VaNorm));
    alpha = acos((Va(1))/VaMagnitude);
else
    alpha = 0;
end

phiA = atan2(Va(2),Va(3));

end

== matlab function elementsLibrary/Earthv1/MATLAB Function ==
  data: altitude input; temperature output; pressure output; density output
function [temperature, pressure, density] = calcTPRho(altitude)

if(altitude < 11000)
    temperature = 15.04 - 0.00649*altitude;
    pressure = 101.29*((temperature + 273.1)/(288.08))^(5.256);
    density = pressure/(0.2896*(temperature + 273.1));
elseif(altitude >= 11000 && altitude < 25000)
    temperature = -56.46;
    pressure = 22.65*exp(1.73 - 0.000157*altitude);
    density = pressure/(0.2896*(temperature + 273.1));
else
    temperature = -131.21 + 0.00299*altitude;
    pressure = 2.488*((temperature + 273.1)/(216.6));
    density = pressure/(0.2896*(temperature + 273.1));
end

end

== matlab function elementsLibrary/nitrousTank1/sat_n20_temperature_calc ==
  data: oldTemperature input; temperature output; specHtCp input; enthVap input; liquidMass input; vapourizedMass input; deltaTemp output
function [temperature, deltaTemp] = nox_temp(oldTemperature, specHtCp, ...
                                             enthVap, liquidMass,...
                                             vapourizedMass)

if(liquidMass >= 0.01)
    % calculate 'differential' of temperature
    deltaQ = vapourizedMass * enthVap;
    deltaTemp = -(deltaQ / (specHtCp * liquidMass));
    
    % calculate new temperature based on old temperature and deltaT
    temperature = oldTemperature + deltaTemp;

else
    deltaTemp = 0;
    temperature = oldTemperature + deltaTemp;
end
                            
end

== matlab function elementsLibrary/nitrousTank1/output_selection1 ==
  data: n2o_sat_pressure input; n2o_sel_p output; liquidMass input; vapMass input; satLiqDens input; satLiqTemp input; vapDens input; vapTemp input; n2o_sel_rho output; n2o_sel_Temp output; vapPres input
function [n2o_sel_p, n2o_sel_rho, n2o_sel_Temp] = ...
    outSelect(n2o_sat_pressure, liquidMass, vapMass,...
              satLiqDens, satLiqTemp,...
              vapDens, vapTemp, vapPres)

    if (liquidMass ~= 0)
        n2o_sel_p = n2o_sat_pressure;
        n2o_sel_rho = satLiqDens;
        n2o_sel_Temp = satLiqTemp;
    else
        n2o_sel_p = vapPres;
        n2o_sel_rho = vapDens;
        n2o_sel_Temp = vapTemp;
    end
end

== matlab function elementsLibrary/nitrousTank1/nox_blowdown ==
  data: massGone input; liquidDens input; vapDens input; tankPressure input; oldLiquidMass input; oldVapourizedMass input; timeStep parameter; vapMass output; liquidMass output; initOxiMass parameter; tankVolume parameter; massProp output; vapourizedMass output; n2o_pCrit parameter; n2o_rhoCrit parameter; n2o_tCrit parameter; n2o_ZCrit parameter; n2o_gamma parameter; initLiqMass parameter; vapTemp input; vapourDens output; vapourTemp output; vapourPres output
function [vapMass, liquidMass, massProp, vapourizedMass, vapourDens, vapourTemp, vapourPres] = ...
    noxBlowdown (massGone, liquidDens, vapDens, ...
                 tankPressure, oldLiquidMass, oldVapourizedMass,...
                 timeStep, initOxiMass, tankVolume,...
                 n2o_pCrit, n2o_rhoCrit, n2o_tCrit,...
                 n2o_ZCrit, n2o_gamma, initLiqMass, vapTemp)

% When oldLiquidMass >= 0.1, run dynamics for liquid blowdown
% When oldLiquidMass < 0.1, no more liquid n2o in tank - run vapour
% blowdown.
%
persistent initVapDens
persistent initVapTemp
persistent initVapPres
persistent initVapMass
persistent initGuessZ

if isempty(initVapDens) || isempty(initVapTemp) || isempty(initVapPres) || isempty(initVapMass) ||isempty(initGuessZ)
    initVapDens = 1;
    initVapTemp = 1;
    initVapPres = 1;
    initVapMass = 1;
    initGuessZ = 1;
end

% This could be done better, but it will work for this purpose.
if(oldLiquidMass >= 0.01)
    % calculate current mass of nitrous in tank (liquid and gas)
    massProp = initOxiMass - massGone;

    % Assume the reduction of mass is completely due to liquid leaving the 
    % tank. ie. no vapour leaving tank
    liquidMassNaive = initLiqMass - massGone;
        
    % calculate next liquid mass and vapour mass
    volPerMassRatio = (1.0/liquidDens) - (1.0/vapDens);
    liquidMass = (tankVolume - (massProp/vapDens))/volPerMassRatio;
    vapMass = massProp - liquidMass;
    
    if liquidMass > liquidMassNaive
        liquidMass = liquidMassNaive;
    end
    
    currVapourizedMass = liquidMassNaive - liquidMass;

    % adjust for finite time required for boiling (ie. not instantaneous)
    % add a 1st-order time lag (of 0.15 seconds) to aid n umerical stability
    tc = timeStep/0.15;
    vapourizedMass = tc*(currVapourizedMass - oldVapourizedMass) + ...
                     oldVapourizedMass;
    
    % during saturation blowdown (liquid still in tank), the density and
    % temperature of the vapour is calculated by the lookup tables outside
    % this function
    vapourDens = vapDens;
    vapourTemp = vapTemp;
    vapourPres = tankPressure;
        
    initVapDens = liquidDens;
    initVapTemp = vapTemp + 273.15;     %converted to kelvin
    initVapPres = tankPressure;
    initVapMass = vapMass;
    initGuessZ = interp1([0, n2o_pCrit],[1, n2o_ZCrit], tankPressure);

else
    % calculate current mass of nitrous in tank (liquid and gas)
    massProp = initOxiMass - massGone;
    
    vapourizedMass = 0;
    liquidMass = 0;
    
    % Assume the reduction of mass is completely due to Vapour leaving the 
    % tank ie. no liquid leaving tank - because no liquid present in tank 
    % for this case
    vapMass = massProp;
    
    currentGuessZ = interp1([0, n2o_pCrit],[1, n2o_ZCrit], tankPressure);
    vapourTemp = vapTemp;           %dummy assignment to trick simulink
    vapourPres = tankPressure;      %dummy assignment to trick simulink
    
    step = 1.0/0.9;
    oldAim = 2;
    Aim = 0;
    
    % Force the loop to execute at least once (this could probably be more
    % elegant)
    loopCond = true;
    
    while (loopCond)
        
        % TODO: get rid of all the bobs, we don't need to use temporary
        %       variables in that way (and if we do, we should name them 
        %       properly)
        bob = n2o_gamma - 1.0; 
        vapourTemp = initVapTemp * ((vapMass * currentGuessZ) / (initVapMass * initGuessZ))^bob;
        bob = n2o_gamma / (n2o_gamma - 1.0);     
        vapourPres = initVapPres * (vapourTemp / initVapTemp)^bob;     
        currentZ = interp1([0, n2o_pCrit],[1, n2o_ZCrit], vapourPres);
        oldAim = Aim;
     
        if (currentGuessZ < currentZ)
            currentGuessZ = currentGuessZ * step;
            Aim = 1;
        else
            currentGuessZ = currentGuessZ / step;
            Aim = -1;
        end
     
        if (Aim == -(oldAim))
            step = sqrt(step);
        end
        
        loopCond = ((currentGuessZ / currentZ) > 1.000001 ||...
                   ((currentGuessZ / currentZ) < (1.0 / 1.000001)));
    
    end
    
    %TODO: No more bobs!
    bob = 1.0 / (n2o_gamma - 1.0); %noxGamma is a constant
    vapourDens = initVapDens * (vapourTemp / initVapTemp)^bob;
    
    vapourTemp = vapourTemp - 273.15;
    
    % clamp down after vapour has run out. This could be done more
    % elegantly (it could be in an else statement of the overall if/else 
    % block in this function)
    if (vapMass < 0.01)
        vapMass = 0;
        massProp = 0;
    end

end

    


end

== matlab function elementsLibrary/barrowmanExt/Coefficent of drag 0 AOA/Pressure Drag Coefficient/MATLAB Function ==
  data: mach input; stagD output
function stagD = getStagDrag(mach)
    if(mach<=1)
        stagD = 1+((mach^2)/4)+((mach^4)/40);
    else
        stagD = 1.84-(0.76/mach^2)+(0.166/mach^4)+(0.035/mach^6);
    end
    stagD=0.85*stagD;
end

== matlab function elementsLibrary/barrowmanExt/MATLAB Function ==
  data: airSpeed input; AOA output; rollAngle output
function [AOA,rollAngle]  = calcAOA(airSpeed)

airSpeed_Mag = (sqrt((airSpeed(1)).^2 + (airSpeed(2)).^2 + (airSpeed(3)).^2)); 

if(airSpeed_Mag>0.01)
    AOA = acos((airSpeed(1))./(airSpeed_Mag));
else
    AOA = 0;
end
rollAngle = atan2(airSpeed(2),airSpeed(3));
end

== matlab function elementsLibrary/barrowmanExt/calcKCoeffs ==
  data: mach input; k1 output; spHt input; k2 output; k3 output
function [k1,k2,k3] = calcKCoeffs(mach,spHt)

b=sqrt(abs((mach^2)-1));

k1=2/b;

k2=((spHt+1)*(mach^4)-4*b^2)/(4*b^4);

k3=((spHt+1)*(mach^8)+(2*spHt^2-7*spHt-5)*mach^6+10*(spHt+1)*mach^4+8)/(6*b^7);

== matlab function elementsLibrary/barrowmanExt/Coefficent of drag 0 AOA/Friction Drag Coefficient/MATLAB Function1 ==
  data: mach input; RE input; Cf output
function Cf  = getCf(mach, RE)
%All roughness corrections ignored since roughness data is unavailable
%Try with and without perfect finish to see which is more reasonable
perfectFinish = 1;
c1=1.0;
c2=1.0;

if(perfectFinish == 1)
    if(RE<1e4)
        Cf=1.33e-2;
    elseif(RE<5.39e5)
        Cf=1.328./(sqrt(RE));
    else
        Cf=1.0./(((1.5.*log(RE)-5.6).^2)-1700./RE);
    end
    
    if(mach<1.1&&RE>1e6)
        if(RE<3e6)
            c1=1.0-0.1.*(mach.^2)*(RE-1e6)./2e6;
        else
            c1=1-0.1.*mach.^2;
        end
    end
    
    if(mach>0.9&&RE>1e6)
        if(RE<3e6)
            c2=1.0+(1.0./((1.0+0.045.*(mach.^2)).^0.25)-1).*(RE-1e6)./2e6;
        else
            c2=1.0/((1.0+0.045*(mach.^2)).^0.25);
        end
    end
    
    if(mach<0.9)
        Cf=Cf*c1;
    elseif(mach<1.1)
        Cf=Cf*(c2*(mach-0.9)/0.2+c1*(1.1-mach)/ 0.2);
    else
        Cf=Cf*c2;
    end
else
    if(RE<1e4)
        Cf=1.48e-2;
    else
        Cf=1.0/(1.5*log(RE)-5.6).^2;
    end
    if(mach<1.1)
        c1=1.0-0.1*mach.^2;
    end
    if(mach>0.9)
        c2=1/(1+0.15*(mach.^2)).^0.58;
    end
    if(mach<0.9)
        Cf=Cf*c1;
    elseif(mach<1.1)
        Cf=Cf*(c2*(mach-0.9)/0.2+c1*(1.1-mach)/0.2);
    else
        Cf=Cf*c2;
    end
end

== matlab function elementsLibrary/barrowmanExt/Coefficent of drag 0 AOA/Friction Drag Coefficient/MATLAB Function2 ==
  data: mach input; RE input; Cf output
function Cf  = getCf(mach, RE)
%All roughness corrections ignored since roughness data is unavailable
%Try with and without perfect finish to see which is more reasonable
perfectFinish = 1;
c1=1.0;
c2=1.0;

if(perfectFinish == 1)
    if(RE<1e4)
        Cf=1.33e-2;
    elseif(RE<5.39e5)
        Cf=1.328./(sqrt(RE));
    else
        Cf=1.0./(((1.5.*log(RE)-5.6).^2)-1700./RE);
    end
    
    if(mach<1.1&&RE>1e6)
        if(RE<3e6)
            c1=1.0-0.1.*(mach.^2)*(RE-1e6)./2e6;
        else
            c1=1-0.1.*mach.^2;
        end
    end
    
    if(mach>0.9&&RE>1e6)
        if(RE<3e6)
            c2=1.0+(1.0./((1.0+0.045.*(mach.^2)).^0.25)-1).*(RE-1e6)./2e6;
        else
            c2=1.0/((1.0+0.045*(mach.^2)).^0.25);
        end
    end
    
    if(mach<0.9)
        Cf=Cf*c1;
    elseif(mach<1.1)
        Cf=Cf*(c2*(mach-0.9)/0.2+c1*(1.1-mach)/ 0.2);
    else
        Cf=Cf*c2;
    end
else
    if(RE<1e4)
        Cf=1.48e-2;
    else
        Cf=1.0/(1.5*log(RE)-5.6).^2;
    end
    if(mach<1.1)
        c1=1.0-0.1*mach.^2;
    end
    if(mach>0.9)
        c2=1/(1+0.15*(mach.^2)).^0.58;
    end
    if(mach<0.9)
        Cf=Cf*c1;
    elseif(mach<1.1)
        Cf=Cf*(c2*(mach-0.9)/0.2+c1*(1.1-mach)/0.2);
    else
        Cf=Cf*c2;
    end
end

== matlab function elementsLibrary/barrowmanExt/Coefficent of drag 0 AOA/Base Drag Coefficient/MATLAB Function1 ==
  data: mach input; baseD output
function baseD = getBaseD(mach)
    if(mach<=1)
        baseD = 0.12+0.13*mach^2;
    else
        baseD = 0.25/mach;
    end

== matlab function elementsLibrary/Ascentv2/Rotational/quaternion_evolution/Calculate Euler Triplet from Quaternion ==
  data: Quaternions input; euler_angles output
function euler_angles = qToEuler(Quaternions)

q0 = Quaternions(1);
q1 = Quaternions(2);
q2 = Quaternions(3);
q3 = Quaternions(4);

Phi = atan2(2.*(q0.*q1 + q2.*q3), (q0^2)-(q1^2)-(q2^2)+(q3^2));
Theta = asin(complex(2.*(q0.*q2 - q3.*q1)));
Psi = atan2(2.*(q0.*q3 +q1.*q2), (q0^2)+(q1^2)-(q2^2)-(q3^2));

euler_angles = [Phi; Theta; Psi];

== matlab function elementsLibrary/Ascentv2/Rotational/quaternion_evolution/Calculate Rate of Change of Quaternions ==
  data: angularVelocities_B input; ddt_Quaternions output; Quaternions input
function ddt_Quaternions = ddtQuaternions(angularVelocities_B, Quaternions)

%const correction factor [experimental]
k = 0; 

lambda = 1 - (Quaternions(1)^2 +...
              Quaternions(2)^2 +...
              Quaternions(3)^2 +...
              Quaternions(4)^2);

p = angularVelocities_B(1);
q = angularVelocities_B(2);
r = angularVelocities_B(3);

qT = [0 -p -q -r; p 0 r -q; q -r 0 p; r q -p 0];

ddt_Quaternions = 0.5*qT*Quaternions + (k*lambda)*Quaternions;
